simulink model "Computer_rel"  (R2018b)
settings: configuration reference "Configuration" (kept outside this file)
model workspace (MATLAB code in the model file):
  | CON = Simulink.Parameter;
  | CON.DataType = 'Bus: Bus_CON';
  | CON.Value = Simulink.Bus.createMATLABStruct('Bus_CON');
undefined symbols (not defined in the file): computer_dt
settings Model: ParameterArgumentNames=CON  OrderedModelArguments=off  Creator=Ethan  LastModifiedBy=Ethan
settings ConfigSetRef: SourceLocation=Base Workspace

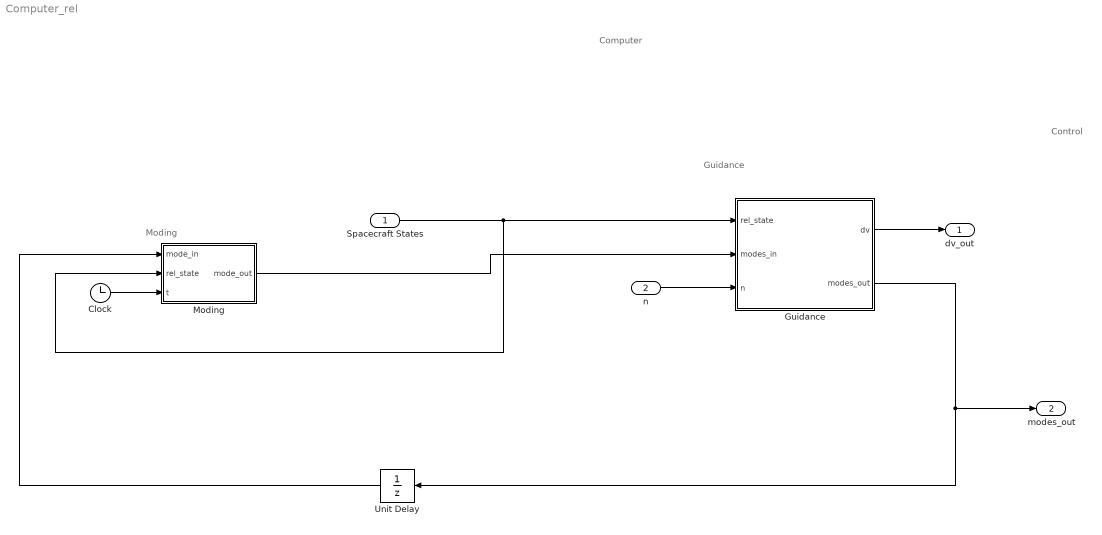
== system Computer_rel ==
  note: Computer
  note: Moding
  note: Control
  note: Guidance
  Spacecraft States : Inport  PortDimensions=6
  n : Inport  Port=2  PortDimensions=1
  Clock : Clock
  Guidance : MATLAB Function  TreatAsAtomicUnit=on  SystemSampleTime=computer_dt
  Moding : MATLAB Function  TreatAsAtomicUnit=on  SystemSampleTime=computer_dt
  Unit Delay : UnitDelay  SampleTime=-1
  dv_out : Outport  PortDimensions=3
  modes_out : Outport  Port=2  OutDataTypeStr=Bus: Bus_modes
  wires:
  Spacecraft States/1 -> Moding/2(rel_state), Guidance/1(rel_state)
  Guidance/1(dv) -> dv_out/1
  Clock/1 -> Moding/3(t)
  Moding/1(mode_out) -> Guidance/2(modes_in)
  Guidance/2(modes_out) -> modes_out/1, Unit Delay/1
  Unit Delay/1 -> Moding/1(mode_in)
  n/1 -> Guidance/3(n)

== matlab function Computer_rel/Guidance ==
  data: rel_state input; modes_in input Bus: Bus_modes; n input; dv output; modes_out output Bus: Bus_modes
function [dv, modes_out] = guid_bound_motion(rel_state, modes_in, n)
modes_out = modes_in;
dv = zeros(3, 1);


persistent dv_old
if isempty(dv_old)
    dv_old = zeros(3, 1);
end
desired_pos = [1, -15, 0]';

if modes_in.guid == 1
    v_desired = -2 * n * rel_state(1);
    dv = [0;v_desired;0] - rel_state(4:6);
    modes_in.guid = 2;
    
elseif modes_out.guid == 3
    w = 80 * pi / 180;
    t = w / n;
    dv = cw_1burn(n, t, rel_state, desired_pos);
    modes_in.guid = 4;
elseif modes_out.guid == 5
    dv = circ_burn(rel_state, n);
end
modes_out = modes_in;
dv_old = dv;
dv = zeros(3, 1);
end

== matlab function Computer_rel/Moding ==
  data: mode_in input Bus: Bus_modes; rel_state input; mode_out output Bus: Bus_modes; t input
function mode_out = moding(mode_in, rel_state,t)

mode_out  = mode_in; 
persistent tig_time
if isempty(tig_time)
    tig_time = 0;
end
desired_pos = [1, 0, 0]';
if rel_state ~= zeros(6, 1)
    if rel_state(2) < 0.5 && mode_in.guid == 10
        mode_out.guid = 1;
        tig_time = t;
    elseif mode_in.guid == 0 && (t - tig_time) > 100
        mode_out.guid = 3;   
    elseif mode_in.guid == 4 && abs(rel_state(1) - desired_pos(1))<0.010
        mode_out.guid = 5;
    end
    
end
